simulink model "problem2"  (R2020b)
settings: Solver=VariableStepAuto  StartTime=0.0  StopTime=10.0  RelTol=1e-3
undefined symbols (not defined in the file): DiscIntNeverNeededParam
libraries: simulink x1
settings Model: Creator=Shree  LastModifiedBy=Shree

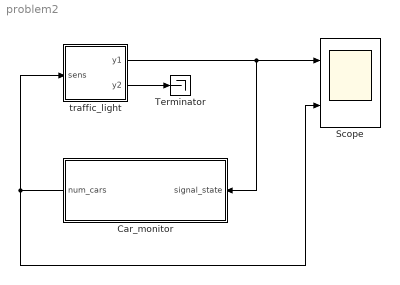
== system problem2 ==
  Car_monitor : Subsystem
  Scope : Scope  NumInputPorts=2
  Terminator : Terminator
  traffic_light : Stateflow chart  TreatAsAtomicUnit=on
  wires:
  traffic_light/2(y2) -> Terminator/1
  traffic_light/1(y1) -> Car_monitor/1(signal_state), Scope/1
  Car_monitor/1(num_cars) -> traffic_light/1(sens), Scope/2

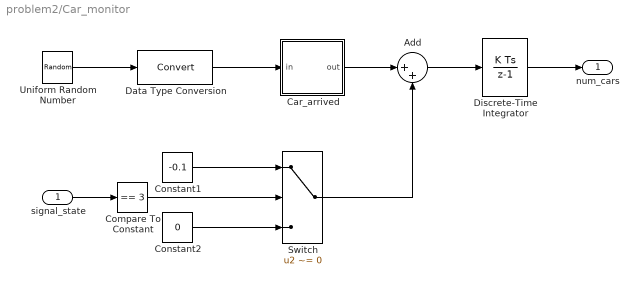
== system problem2/Car_monitor ==
  signal_state : Inport
  Add : Sum  Inputs=|++
  Car_arrived : Stateflow chart  TreatAsAtomicUnit=on
  Compare To Constant : simulink/Logic and Bit Operations/Compare To Constant  relop===  const=3  OutDataTypeStr=boolean  ZeroCross=off
  Constant1 : Constant  Value=-0.1
  Constant2 : Constant  Value=0
  Data Type Conversion : DataTypeConversion
  Discrete-Time Integrator : DiscreteIntegrator  SampleTime=-1  LimitOutput=on  LowerSaturationLimit=0  ICPrevOutput=DiscIntNeverNeededParam  ICPrevScaledInput=DiscIntNeverNeededParam
  Switch : Switch  Criteria=u2 ~= 0
  Uniform Random Number : UniformRandomNumber  Minimum=0  Maximum=100  Seed=177836  SampleTime=0
  num_cars : Outport  VectorParamsAs1DForOutWhenUnconnected=off
  wires:
  Add/1 -> Discrete-Time Integrator/1
  Car_arrived/1(out) -> Add/1
  Discrete-Time Integrator/1 -> num_cars/1
  Data Type Conversion/1 -> Car_arrived/1(in)
  Compare To Constant/1 -> Switch/2
  Constant1/1 -> Switch/1
  Switch/1 -> Add/2
  Constant2/1 -> Switch/3
  Uniform Random Number/1 -> Data Type Conversion/1
  signal_state/1 -> Compare To Constant/1

== stateflow chart problem2/traffic_light ==
  settings: stateMachineType=MOORE_MACHINE  initializeOutput=1
  state Stop1
    y1 = RED;
    y2 = GREEN;
  state StopForTraffic1
    y1 = RED;
    y2 = GREEN;
  state StopToGo1
    y1 = RED;
    y2 = YELLOW;
  state GoToStop1
    y1 = YELLOW;
    y2 = RED;
  state Go1
    y1 = GREEN;
    y2 = RED;
  (default) -> Stop1
  StopForTraffic1 -> StopToGo1 : [sens]
  Stop1 -> StopForTraffic1 : after(20,tick)
  GoToStop1 -> Stop1 : after (3,tick)
  StopToGo1 -> Go1 : after(3,tick)
  Go1 -> GoToStop1 : after(10,tick)
  data: sens input double; y1 output double; y2 output double; GREEN constant double =3; RED constant uint8 =1; YELLOW constant double =2

== stateflow chart problem2/Car_monitor/Car_arrived ==
  (default) -> (junction 2) : {out = in > 98;}
  data: in input int8; out output double
